simulink model "Goto_Tag_Visibility"  (R2014a)
settings: Solver=FixedStepDiscrete  StartTime=0.0  StopTime=10.0  FixedStep=0.1  RelTol=1e-3
settings Model: BufferReuse=off  Creator=kohei-y  LastModifiedBy=ts1413
settings OptimizationCC: BlockReduction=off  OptimizeBlockIOStorage=off  BufferReuse=off  GlobalBufferReuse=off  ExpressionFolding=off  LocalBlockOutputs=off  OptimizeModelRefInitCode=on  LifeSpan=1
settings RTWCC: SystemTargetFile=ert.tlc  GenCodeOnly=on  TemplateMakefile=ert_default_tmf  Description=Embedded Coder  ProcessScript=ert_make_rtw_hook  IncludeHyperlinkInReport=on
settings CodeAppCC: IgnoreCustomStorageClasses=off
settings ERTTargetCC: ParMdlRefBuildCompliant=on  CompOptLevelCompliant=on  ConcurrentExecutionCompliant=on  ERTFirstTimeCompliant=on  ModelStepFunctionPrototypeControlCompliant=on  CPPClassGenCompliant=on  InlinedParameterPlacement=Hierarchical  ERTCustomFileTemplate=example_file_process.tlc

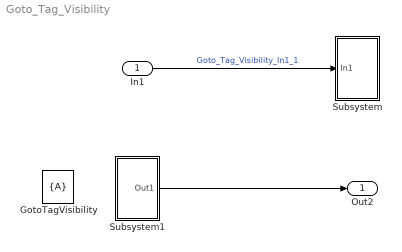
== system Goto_Tag_Visibility ==
  In1 : Inport
  GotoTagVisibility : GotoTagVisibility
  Subsystem : Subsystem
  Subsystem1 : Subsystem
  Out2 : Outport
  wires:
  In1/1 -> Subsystem/1(In1)  "Goto_Tag_Visibility_In1_1"
  Subsystem1/1(Out1) -> Out2/1

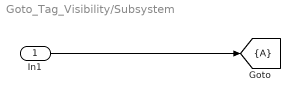
== system Goto_Tag_Visibility/Subsystem ==
  In1 : Inport
  tag scope: A=scoped
  wires:
  In1/1 -> [A]

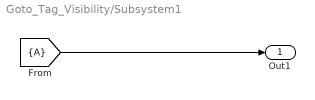
== system Goto_Tag_Visibility/Subsystem1 ==
  Out1 : Outport
  wires:
  [A] -> Out1/1
